simulink model "aerotest"  (R2021b)
settings: Solver=VariableStepAuto  StartTime=0.0  StopTime=10.0  RelTol=1e-3
undefined symbols (not defined in the file or in its folder): admireDB
libraries: simulink_extras x103, simulink x24, aerolibatmos2 x1
(part 2 of 13)

== system aerotest/YawMomentCoefficient/Subsystem ==
  mach_nd : Inport
  CymtotMR1 : Inport  Port=2
  CymtotMR2 : Inport  Port=3
  CymtotMR3 : Inport  Port=4
  CymtotMR4 : Inport  Port=5
  AND : Logic  IconShape=distinctive  AllPortsSameDT=off  OutDataTypeStr=boolean
  AND1 : Logic  IconShape=distinctive  AllPortsSameDT=off  OutDataTypeStr=boolean
  Compare To Constant1 : simulink/Logic and Bit Operations/Compare To Constant  relop=<=  const=0.4  OutDataTypeStr=boolean
  Compare To Constant2 : simulink/Logic and Bit Operations/Compare To Constant  relop=>  const=0.4  OutDataTypeStr=boolean
  Compare To Constant3 : simulink/Logic and Bit Operations/Compare To Constant  relop=<  const=0.5  OutDataTypeStr=boolean
  Compare To Constant4 : simulink/Logic and Bit Operations/Compare To Constant  relop=<=  const=1.4  OutDataTypeStr=boolean
  Compare To Constant5 : simulink/Logic and Bit Operations/Compare To Constant  relop=>=  const=0.5  OutDataTypeStr=boolean
  Switch : Switch  Criteria=u2 ~= 0
  Switch1 : Switch  Criteria=u2 ~= 0
  Switch2 : Switch  Criteria=u2 ~= 0
  Cymtot : Outport
  wires:
  Compare To Constant5/1 -> AND1/1
  Compare To Constant4/1 -> AND1/2
  AND1/1 -> Switch2/2
  CymtotMR4/1 -> Switch2/3
  CymtotMR3/1 -> Switch2/1
  Switch/1 -> Cymtot/1
  Switch2/1 -> Switch1/3
  CymtotMR2/1 -> Switch1/1
  Switch1/1 -> Switch/3
  CymtotMR1/1 -> Switch/1
  AND/1 -> Switch1/2
  Compare To Constant3/1 -> AND/2
  Compare To Constant2/1 -> AND/1
  Compare To Constant1/1 -> Switch/2
  mach_nd/1 -> Compare To Constant1/1, Compare To Constant3/1, Compare To Constant4/1, Compare To Constant5/1, Compare To Constant2/1

== system aerotest/CentripetalForceCoefficient/MachRegion1/Ccbcai ==
  in_bus : Inport
  Bus Selector : BusSelector  OutputSignals=AeroIn_Bus.cai,AeroIn_Bus.angleOfAttack_deg,AeroIn_Bus.angleOfSideslip_deg
  Ccbcai_ : Subsystem
  Ccbcai : Outport
  wires:
  Bus Selector/3 -> Ccbcai_/3(angleOfSideslip_deg)  "<angleOfSideslip_deg>"
  Bus Selector/2 -> Ccbcai_/2(angleOfAttack_deg)  "<angleOfAttack_deg>"
  in_bus/1 -> Bus Selector/1  "in_bus"
  Ccbcai_/1(Ccbcai) -> Ccbcai/1
  Bus Selector/1 -> Ccbcai_/1(CAI)  "<cai>"

== system aerotest/CentripetalForceCoefficient/MachRegion1/Ccbde ==
  in_bus : Inport
  Bus Selector : BusSelector  OutputSignals=AeroIn_Bus.angleOfSideslip_deg,AeroIn_Bus.dEI,AeroIn_Bus.angleOfAttack_deg,eieff,AeroIn_Bus.dEY,eoeff
  Ccbde_ : Subsystem
  Ccbde : Outport
  wires:
  Bus Selector/6 -> Ccbde_/6(eoeff)  "<eoeff>"
  Bus Selector/5 -> Ccbde_/5(dEY)  "<dEY>"
  Bus Selector/4 -> Ccbde_/4(eieff)  "<eieff>"
  Bus Selector/3 -> Ccbde_/3(angleOfAttack_deg)  "<angleOfAttack_deg>"
  Bus Selector/2 -> Ccbde_/2(dEI)  "<dEI>"
  Bus Selector/1 -> Ccbde_/1(angleOfSideslip_deg)  "<angleOfSideslip_deg>"
  Ccbde_/1(Ccbde) -> Ccbde/1
  in_bus/1 -> Bus Selector/1  "in_bus"

== system aerotest/CentripetalForceCoefficient/MachRegion1/Ccbdle ==
  in_bus : Inport
  Bus Selector : BusSelector  OutputSignals=AeroIn_Bus.lef_deg,AeroIn_Bus.angleOfSideslip_deg,AeroIn_Bus.angleOfAttack_deg
  Ccbdle_ : Subsystem
  Ccbdle : Outport
  wires:
  Bus Selector/3 -> Ccbdle_/3(angleOfAttack_deg)  "<angleOfAttack_deg>"
  Bus Selector/2 -> Ccbdle_/2(angleOfSideslip_deg)  "<angleOfSideslip_deg>"
  Bus Selector/1 -> Ccbdle_/1(dLE)  "<lef_deg>"
  Ccbdle_/1(Ccbdle) -> Ccbdle/1
  in_bus/1 -> Bus Selector/1  "in_bus"

== system aerotest/CentripetalForceCoefficient/MachRegion1/Ccbdn ==
  in_bus : Inport
  Bus Selector : BusSelector  OutputSignals=AeroIn_Bus.angleOfSideslip_deg,AeroIn_Bus.dN,AeroIn_Bus.angleOfAttack_deg
  Ccbdn_ : Subsystem
  Ccbdn : Outport
  wires:
  Bus Selector/2 -> Ccbdn_/2(dN)  "<dN>"
  Bus Selector/1 -> Ccbdn_/1(angleOfSideslip_deg)  "<angleOfSideslip_deg>"
  Bus Selector/3 -> Ccbdn_/3(angleOfAttack_deg)  "<angleOfAttack_deg>"
  in_bus/1 -> Bus Selector/1  "in_bus"
  Ccbdn_/1(Ccbdn) -> Ccbdn/1

== system aerotest/CentripetalForceCoefficient/MachRegion1/Ccbeta ==
  in_bus : Inport
  Bus Selector : BusSelector  OutputSignals=AeroIn_Bus.angleOfSideslip_deg,AeroIn_Bus.angleOfAttack_deg,AeroIn_Bus.qacorr,AeroIn_Bus.mach_nd
  Ccbeta_ : Subsystem
  Ccbeta : Outport
  wires:
  Ccbeta_/1(Ccbeta) -> Ccbeta/1
  Bus Selector/4 -> Ccbeta_/4(mach_nd)  "<mach_nd>"
  Bus Selector/3 -> Ccbeta_/3(qacorr)  "<qacorr>"
  Bus Selector/2 -> Ccbeta_/2(angleOfAttack_deg)  "<angleOfAttack_deg>"
  Bus Selector/1 -> Ccbeta_/1(angleOfSideslip_deg)  "<angleOfSideslip_deg>"
  in_bus/1 -> Bus Selector/1  "in_bus"

== system aerotest/CentripetalForceCoefficient/MachRegion1/Ccbetad ==
  in_bus : Inport
  Bus Selector : BusSelector  OutputSignals=AeroIn_Bus.angleOfAttack_deg,AeroIn_Bus.betad
  Ccbetad_ : Subsystem
  Ccbetad : Outport
  wires:
  Bus Selector/2 -> Ccbetad_/2(betad)  "<betad>"
  Bus Selector/1 -> Ccbetad_/1(angleOfAttack_deg)  "<angleOfAttack_deg>"
  in_bus/1 -> Bus Selector/1  "in_bus"
  Ccbetad_/1(Ccbetad) -> Ccbetad/1

== system aerotest/CentripetalForceCoefficient/MachRegion1/Ccblg ==
  in_bus : Inport
  Bus Selector : BusSelector  OutputSignals=AeroIn_Bus.lg_bool,AeroIn_Bus.angleOfAttack_deg,AeroIn_Bus.angleOfSideslip_deg
  Ccblg_ : Subsystem
  Ccblg : Outport
  wires:
  Bus Selector/1 -> Ccblg_/1(dLG)  "<lg_bool>"
  Bus Selector/3 -> Ccblg_/3(angleOfSideslip_deg)  "<angleOfSideslip_deg>"
  Bus Selector/2 -> Ccblg_/2(angleOfAttack_deg)  "<angleOfAttack_deg>"
  in_bus/1 -> Bus Selector/1  "in_bus"
  Ccblg_/1(Ccblg) -> Ccblg/1

== system aerotest/CentripetalForceCoefficient/MachRegion1/Ccdai ==
  in_bus : Inport
  Bus Selector : BusSelector  OutputSignals=AeroIn_Bus.dAI,AeroIn_Bus.angleOfAttack_deg,AeroIn_Bus.dEI,eieff,AeroIn_Bus.qacorr,AeroIn_Bus.mach_nd
  Ccdai_ : Subsystem
  Ccdai : Outport
  wires:
  Bus Selector/1 -> Ccdai_/1(dAI)  "<dAI>"
  Bus Selector/2 -> Ccdai_/2(angleOfAttack_deg)  "<angleOfAttack_deg>"
  Bus Selector/3 -> Ccdai_/3(dEI)  "<dEI>"
  Bus Selector/4 -> Ccdai_/4(eieff)  "<eieff>"
  Bus Selector/5 -> Ccdai_/5(qacorr)  "<qacorr>"
  Bus Selector/6 -> Ccdai_/6(mach_nd)  "<mach_nd>"
  in_bus/1 -> Bus Selector/1  "in_bus"
  Ccdai_/1(Ccdai) -> Ccdai/1

== system aerotest/CentripetalForceCoefficient/MachRegion1/Ccdaib ==
  in_bus : Inport
  Bus Selector : BusSelector  OutputSignals=AeroIn_Bus.angleOfAttack_deg,AeroIn_Bus.dAI,AeroIn_Bus.angleOfSideslip_deg,eieff
  Ccdaib_ : Subsystem
  Ccdaib : Outport
  wires:
  Bus Selector/4 -> Ccdaib_/4(eieff)  "<eieff>"
  Bus Selector/3 -> Ccdaib_/3(angleOfSideslip_deg)  "<angleOfSideslip_deg>"
  Bus Selector/1 -> Ccdaib_/1(angleOfAttack_deg)  "<angleOfAttack_deg>"
  Bus Selector/2 -> Ccdaib_/2(dAI)  "<dAI>"
  Ccdaib_/1(Ccdaib) -> Ccdaib/1
  in_bus/1 -> Bus Selector/1  "in_bus"

== system aerotest/CentripetalForceCoefficient/MachRegion1/Ccday ==
  in_bus : Inport
  Bus Selector : BusSelector  OutputSignals=AeroIn_Bus.dAY,AeroIn_Bus.angleOfAttack_deg,AeroIn_Bus.dEY,eoeff,AeroIn_Bus.qacorr,AeroIn_Bus.mach_nd
  Ccday_ : Subsystem
  Ccday : Outport
  wires:
  Ccday_/1(Ccday) -> Ccday/1
  in_bus/1 -> Bus Selector/1  "in_bus"
  Bus Selector/6 -> Ccday_/6(mach_nd)  "<mach_nd>"
  Bus Selector/5 -> Ccday_/5(qacorr)  "<qacorr>"
  Bus Selector/4 -> Ccday_/4(eoeff)  "<eoeff>"
  Bus Selector/3 -> Ccday_/3(dEY)  "<dEY>"
  Bus Selector/2 -> Ccday_/2(angleOfAttack_deg)  "<angleOfAttack_deg>"
  Bus Selector/1 -> Ccday_/1(dAY)  "<dAY>"

== system aerotest/CentripetalForceCoefficient/MachRegion1/Ccdayb ==
  in_bus : Inport
  Bus Selector : BusSelector  OutputSignals=AeroIn_Bus.angleOfAttack_deg,AeroIn_Bus.dAY,AeroIn_Bus.angleOfSideslip_deg,eoeff
  Ccdayb_ : Subsystem
  Ccdayb : Outport
  wires:
  in_bus/1 -> Bus Selector/1  "in_bus"
  Ccdayb_/1(Ccdayb) -> Ccdayb/1
  Bus Selector/2 -> Ccdayb_/2(dAY)  "<dAY>"
  Bus Selector/1 -> Ccdayb_/1(angleOfAttack_deg)  "<angleOfAttack_deg>"
  Bus Selector/3 -> Ccdayb_/3(angleOfSideslip_deg)  "<angleOfSideslip_deg>"
  Bus Selector/4 -> Ccdayb_/4(eoeff)  "<eoeff>"

== system aerotest/CentripetalForceCoefficient/MachRegion1/Ccdna ==
  in_bus : Inport
  Bus Selector : BusSelector  OutputSignals=AeroIn_Bus.dNE,AeroIn_Bus.angleOfAttack_deg,AeroIn_Bus.dNA
  Ccdna_ : Subsystem
  Ccdna : Outport
  wires:
  Bus Selector/3 -> Ccdna_/3(dNA)  "<dNA>"
  Bus Selector/1 -> Ccdna_/1(dNE)  "<dNE>"
  Bus Selector/2 -> Ccdna_/2(angleOfAttack_deg)  "<angleOfAttack_deg>"
  Ccdna_/1(Ccdna) -> Ccdna/1
  in_bus/1 -> Bus Selector/1  "in_bus"

== system aerotest/CentripetalForceCoefficient/MachRegion1/Ccdr ==
  in_bus : Inport
  Bus Selector : BusSelector  OutputSignals=AeroIn_Bus.angleOfAttack_deg,AeroIn_Bus.rud_deg,AeroIn_Bus.angleOfSideslip_deg,AeroIn_Bus.qacorr,AeroIn_Bus.mach_nd
  Ccdr_ : Subsystem
  Ccdr : Outport
  wires:
  Ccdr_/1(Ccdr) -> Ccdr/1
  Bus Selector/1 -> Ccdr_/1(angleOfAttack_deg)  "<angleOfAttack_deg>"
  Bus Selector/2 -> Ccdr_/2(dR)  "<rud_deg>"
  Bus Selector/3 -> Ccdr_/3(angleOfSideslip_deg)  "<angleOfSideslip_deg>"
  Bus Selector/4 -> Ccdr_/4(qacorr)  "<qacorr>"
  Bus Selector/5 -> Ccdr_/5(mach_nd)  "<mach_nd>"
  in_bus/1 -> Bus Selector/1  "in_bus"

== system aerotest/CentripetalForceCoefficient/MachRegion1/Ccp ==
  in_bus : Inport
  Bus Selector : BusSelector  OutputSignals=AeroIn_Bus.angleOfAttack_deg,AeroIn_Bus.pc
  Ccp_ : Subsystem
  Ccp : Outport
  wires:
  Ccp_/1(Ccp) -> Ccp/1
  in_bus/1 -> Bus Selector/1  "in_bus"
  Bus Selector/1 -> Ccp_/1(angleOfAttack_deg)  "<angleOfAttack_deg>"
  Bus Selector/2 -> Ccp_/2(pc)  "<pc>"

== system aerotest/CentripetalForceCoefficient/MachRegion1/Ccpbeta ==
  in_bus : Inport
  Bus Selector : BusSelector  OutputSignals=AeroIn_Bus.angleOfSideslip_deg,AeroIn_Bus.pc,AeroIn_Bus.angleOfAttack_deg
  Ccpbeta_ : Subsystem
  Ccpbeta : Outport
  wires:
  Bus Selector/3 -> Ccpbeta_/3(angleOfAttack_deg)  "<angleOfAttack_deg>"
  Bus Selector/1 -> Ccpbeta_/1(angleOfSideslip_deg)  "<angleOfSideslip_deg>"
  Bus Selector/2 -> Ccpbeta_/2(pc)  "<pc>"
  in_bus/1 -> Bus Selector/1  "in_bus"
  Ccpbeta_/1(Ccpbeta) -> Ccpbeta/1

== system aerotest/CentripetalForceCoefficient/MachRegion1/Ccr ==
  in_bus : Inport
  Bus Selector : BusSelector  OutputSignals=AeroIn_Bus.dN,AeroIn_Bus.angleOfAttack_deg,AeroIn_Bus.rc
  Ccr_ : Subsystem
  Ccr : Outport
  wires:
  Bus Selector/1 -> Ccr_/1(dN)  "<dN>"
  Bus Selector/3 -> Ccr_/3(rc)  "<rc>"
  Bus Selector/2 -> Ccr_/2(angleOfAttack_deg)  "<angleOfAttack_deg>"
  Ccr_/1(Ccr) -> Ccr/1
  in_bus/1 -> Bus Selector/1  "in_bus"

== system aerotest/CentripetalForceCoefficient/MachRegion1/Ccrbeta ==
  in_bus : Inport
  Bus Selector : BusSelector  OutputSignals=AeroIn_Bus.angleOfSideslip_deg,AeroIn_Bus.angleOfAttack_deg,AeroIn_Bus.rc
  Ccrbeta_ : Subsystem
  Ccrbeta : Outport
  wires:
  Bus Selector/3 -> Ccrbeta_/3(rc)  "<rc>"
  Bus Selector/1 -> Ccrbeta_/1(angleOfSideslip_deg)  "<angleOfSideslip_deg>"
  Bus Selector/2 -> Ccrbeta_/2(angleOfAttack_deg)  "<angleOfAttack_deg>"
  in_bus/1 -> Bus Selector/1  "in_bus"
  Ccrbeta_/1(Ccrbeta) -> Ccrbeta/1

== system aerotest/CentripetalForceCoefficient/MachRegion1/eoeff1 ==
  AeroIn_Bus : Inport
  Bus Selector : BusSelector  OutputSignals=mach_nd
  CCDAYOD_M : Lookup_n-D  NumberOfTableDimensions=1  BreakpointsForDimension1=admireDB.aerodata_asym_ext.CCDAYOD.breakpoints.M  BreakpointsForDimension3=[5, 7]  Table=admireDB.aerodata_asym_ext.CCDAYOD.newTable  ExtrapMethod=Clip  InternalRulePriority=Speed  RndMeth=Simplest  InputSameDT=on
  Constant : Constant
  Sum : Sum  Inputs=-+|
  eoeff : Outport
  eieff : Outport  Port=2
  wires:
  Sum/1 -> eieff/1
  CCDAYOD_M/1 -> eoeff/1, Sum/1
  Constant/1 -> Sum/2
  Bus Selector/1 -> CCDAYOD_M/1  "<mach_nd>"
  AeroIn_Bus/1 -> Bus Selector/1

== system aerotest/CentripetalForceCoefficient/MachRegion2/Ccbcai ==
  in_bus : Inport
  Bus Selector : BusSelector  OutputSignals=AeroIn_Bus.cai,AeroIn_Bus.angleOfAttack_deg,AeroIn_Bus.angleOfSideslip_deg
  Ccbcai_ : Subsystem
  Ccbcai : Outport
  wires:
  Bus Selector/1 -> Ccbcai_/1(cai)  "<cai>"
  Bus Selector/3 -> Ccbcai_/3(angleOfSideslip_deg)  "<angleOfSideslip_deg>"
  Bus Selector/2 -> Ccbcai_/2(angleOfAttack_deg)  "<angleOfAttack_deg>"
  in_bus/1 -> Bus Selector/1  "in_bus"
  Ccbcai_/1(Ccbcai) -> Ccbcai/1

== system aerotest/CentripetalForceCoefficient/MachRegion2/Ccbde ==
  in_bus : Inport
  Bus Selector : BusSelector  OutputSignals=AeroIn_Bus.angleOfAttack_deg,AeroIn_Bus.dEI,AeroIn_Bus.angleOfSideslip_deg,eieff,AeroIn_Bus.dEY,eoeff
  Ccbde_ : Subsystem
  Ccbde : Outport
  wires:
  Bus Selector/1 -> Ccbde_/1(angleOfAttack_deg)  "<angleOfAttack_deg>"
  Bus Selector/2 -> Ccbde_/2(dEI)  "<dEI>"
  Bus Selector/3 -> Ccbde_/3(angleOfSideslip_deg)  "<angleOfSideslip_deg>"
  Bus Selector/4 -> Ccbde_/4(eieff)  "<eieff>"
  Bus Selector/5 -> Ccbde_/5(dEY)  "<dEY>"
  Bus Selector/6 -> Ccbde_/6(eoeff)  "<eoeff>"
  Ccbde_/1(Ccbde) -> Ccbde/1
  in_bus/1 -> Bus Selector/1  "in_bus"

== system aerotest/CentripetalForceCoefficient/MachRegion2/Ccbdle ==
  in_bus : Inport
  Bus Selector : BusSelector  OutputSignals=AeroIn_Bus.angleOfAttack_deg,AeroIn_Bus.angleOfSideslip_deg,AeroIn_Bus.lef_deg,AeroIn_Bus.tflow,AeroIn_Bus.tfhigh
  Ccbdle_ : Subsystem
  Ccbdle : Outport
  wires:
  Bus Selector/5 -> Ccbdle_/5(tfhigh)  "<tfhigh>"
  Bus Selector/4 -> Ccbdle_/4(tflow)  "<tflow>"
  Bus Selector/3 -> Ccbdle_/3(dLE)  "<lef_deg>"
  Bus Selector/2 -> Ccbdle_/2(angleOfSideslip_deg)  "<angleOfSideslip_deg>"
  Bus Selector/1 -> Ccbdle_/1(angleOfAttack_deg)  "<angleOfAttack_deg>"
  Ccbdle_/1(Ccbdle) -> Ccbdle/1
  in_bus/1 -> Bus Selector/1  "in_bus"

== system aerotest/CentripetalForceCoefficient/MachRegion2/Ccbdn ==
  in_bus : Inport
  Bus Selector : BusSelector  OutputSignals=AeroIn_Bus.angleOfAttack_deg,AeroIn_Bus.dN,AeroIn_Bus.angleOfSideslip_deg
  Ccbdn_ : Subsystem
  Ccbdn : Outport
  wires:
  Bus Selector/1 -> Ccbdn_/1(angleOfAttack_deg)  "<angleOfAttack_deg>"
  Bus Selector/2 -> Ccbdn_/2(dN)  "<dN>"
  Bus Selector/3 -> Ccbdn_/3(angleOfSideslip_deg)  "<angleOfSideslip_deg>"
  in_bus/1 -> Bus Selector/1  "in_bus"
  Ccbdn_/1(Ccbdn) -> Ccbdn/1

== system aerotest/CentripetalForceCoefficient/MachRegion2/Ccbeta ==
  in_bus : Inport
  Bus Selector : BusSelector  OutputSignals=AeroIn_Bus.angleOfSideslip_deg,AeroIn_Bus.angleOfAttack_deg,AeroIn_Bus.tflow,AeroIn_Bus.tfhigh,AeroIn_Bus.qacorr,AeroIn_Bus.mach_nd
  Ccbeta_ : Subsystem
  Ccbeta : Outport
  wires:
  Bus Selector/6 -> Ccbeta_/6(mach_nd)  "<mach_nd>"
  Bus Selector/5 -> Ccbeta_/5(qacorr)  "<qacorr>"
  Bus Selector/4 -> Ccbeta_/4(tfhigh)  "<tfhigh>"
  Bus Selector/3 -> Ccbeta_/3(tflow)  "<tflow>"
  Bus Selector/2 -> Ccbeta_/2(angleOfAttack_deg)  "<angleOfAttack_deg>"
  Bus Selector/1 -> Ccbeta_/1(angleOfSideslip_deg)  "<angleOfSideslip_deg>"
  Ccbeta_/1(CCbeta) -> Ccbeta/1
  in_bus/1 -> Bus Selector/1  "in_bus"

== system aerotest/CentripetalForceCoefficient/MachRegion2/Ccbetad ==
  in_bus : Inport
  Bus Selector : BusSelector  OutputSignals=AeroIn_Bus.angleOfAttack_deg,AeroIn_Bus.tflow,AeroIn_Bus.betad,AeroIn_Bus.tfhigh
  CCbetad_ : Subsystem
  Ccbetad : Outport
  wires:
  Bus Selector/4 -> CCbetad_/4(tfhigh)  "<tfhigh>"
  Bus Selector/3 -> CCbetad_/3(betad)  "<betad>"
  Bus Selector/1 -> CCbetad_/1(angleOfAttack_deg)  "<angleOfAttack_deg>"
  Bus Selector/2 -> CCbetad_/2(tflow)  "<tflow>"
  CCbetad_/1(CCbetad) -> Ccbetad/1
  in_bus/1 -> Bus Selector/1  "in_bus"

== system aerotest/CentripetalForceCoefficient/MachRegion2/Ccblg ==
  in_bus : Inport
  Bus Selector : BusSelector  OutputSignals=AeroIn_Bus.lg_bool,AeroIn_Bus.angleOfAttack_deg,AeroIn_Bus.angleOfSideslip_deg
  Ccblg_ : Subsystem
  Ccblg : Outport
  wires:
  Bus Selector/1 -> Ccblg_/1(ldg)  "<lg_bool>"
  Bus Selector/3 -> Ccblg_/3(angleOfSideslip_deg)  "<angleOfSideslip_deg>"
  Bus Selector/2 -> Ccblg_/2(angleOfAttack_deg)  "<angleOfAttack_deg>"
  in_bus/1 -> Bus Selector/1  "in_bus"
  Ccblg_/1(Ccblg) -> Ccblg/1

== system aerotest/CentripetalForceCoefficient/MachRegion2/Ccdai ==
  in_bus : Inport
  Bus Selector : BusSelector  OutputSignals=AeroIn_Bus.dAI,AeroIn_Bus.angleOfAttack_deg,AeroIn_Bus.dEI,AeroIn_Bus.qacorr,AeroIn_Bus.mach_nd,AeroIn_Bus.tflow,AeroIn_Bus.tfhigh,eieff
  Ccdai_ : Subsystem
  Ccdai : Outport
  wires:
  Bus Selector/8 -> Ccdai_/8(eieff)  "<eieff>"
  Bus Selector/7 -> Ccdai_/7(tfhigh)  "<tfhigh>"
  Bus Selector/6 -> Ccdai_/6(tflow)  "<tflow>"
  Bus Selector/5 -> Ccdai_/5(mach_nd)  "<mach_nd>"
  Bus Selector/4 -> Ccdai_/4(qacorr)  "<qacorr>"
  Bus Selector/3 -> Ccdai_/3(dEI)  "<dEI>"
  Bus Selector/2 -> Ccdai_/2(angleOfAttack_deg)  "<angleOfAttack_deg>"
  Bus Selector/1 -> Ccdai_/1(dAI)  "<dAI>"
  in_bus/1 -> Bus Selector/1  "in_bus"
  Ccdai_/1(Ccdai) -> Ccdai/1

== system aerotest/CentripetalForceCoefficient/MachRegion2/Ccdaib ==
  in_bus : Inport
  Bus Selector : BusSelector  OutputSignals=AeroIn_Bus.angleOfAttack_deg,AeroIn_Bus.dAI,AeroIn_Bus.angleOfSideslip_deg,AeroIn_Bus.tflow,eieff
  Ccdaib_ : Subsystem
  Ccdaib : Outport
  wires:
  Bus Selector/5 -> Ccdaib_/5(eieff)  "<eieff>"
  Bus Selector/4 -> Ccdaib_/4(tflow)  "<tflow>"
  Bus Selector/3 -> Ccdaib_/3(angleOfSideslip_deg)  "<angleOfSideslip_deg>"
  Bus Selector/2 -> Ccdaib_/2(dAI)  "<dAI>"
  Bus Selector/1 -> Ccdaib_/1(angleOfAttack_deg)  "<angleOfAttack_deg>"
  Ccdaib_/1(Ccdaib) -> Ccdaib/1
  in_bus/1 -> Bus Selector/1  "in_bus"

== system aerotest/CentripetalForceCoefficient/MachRegion2/Ccday ==
  in_bus : Inport
  Bus Selector : BusSelector  OutputSignals=AeroIn_Bus.dAY,AeroIn_Bus.angleOfAttack_deg,AeroIn_Bus.dEY,AeroIn_Bus.qacorr,AeroIn_Bus.mach_nd,AeroIn_Bus.tflow,AeroIn_Bus.tfhigh,eoeff
  Ccday_ : Subsystem
  Ccday : Outport
  wires:
  Bus Selector/8 -> Ccday_/8(eoeff)  "<eoeff>"
  Bus Selector/7 -> Ccday_/7(tfhigh)  "<tfhigh>"
  Bus Selector/6 -> Ccday_/6(tflow)  "<tflow>"
  Bus Selector/5 -> Ccday_/5(mach_nd)  "<mach_nd>"
  Bus Selector/4 -> Ccday_/4(qacorr)  "<qacorr>"
  Bus Selector/3 -> Ccday_/3(dEY)  "<dEY>"
  Bus Selector/2 -> Ccday_/2(angleOfAttack_deg)  "<angleOfAttack_deg>"
  Bus Selector/1 -> Ccday_/1(dAY)  "<dAY>"
  in_bus/1 -> Bus Selector/1  "in_bus"
  Ccday_/1(Ccday) -> Ccday/1

== system aerotest/CentripetalForceCoefficient/MachRegion2/Ccdayb ==
  in_bus : Inport
  Bus Selector : BusSelector  OutputSignals=AeroIn_Bus.angleOfAttack_deg,AeroIn_Bus.dAY,AeroIn_Bus.angleOfSideslip_deg,AeroIn_Bus.tflow,eoeff
  Ccdayb_ : Subsystem
  Ccdayb : Outport
  wires:
  Bus Selector/1 -> Ccdayb_/1(angleOfAttack_deg)  "<angleOfAttack_deg>"
  Bus Selector/2 -> Ccdayb_/2(dAY)  "<dAY>"
  Bus Selector/3 -> Ccdayb_/3(angleOfSideslip_deg)  "<angleOfSideslip_deg>"
  Bus Selector/4 -> Ccdayb_/4(tflow)  "<tflow>"
  Bus Selector/5 -> Ccdayb_/5(eoeff)  "<eoeff>"
  Ccdayb_/1(Ccdaib) -> Ccdayb/1
  in_bus/1 -> Bus Selector/1  "in_bus"

== system aerotest/CentripetalForceCoefficient/MachRegion2/Ccdna ==
  in_bus : Inport
  Bus Selector : BusSelector  OutputSignals=AeroIn_Bus.dNE,AeroIn_Bus.angleOfAttack_deg,AeroIn_Bus.tflow,AeroIn_Bus.tfhigh,AeroIn_Bus.dNA
  Ccdna_ : Subsystem
  Ccdna : Outport
  wires:
  Bus Selector/5 -> Ccdna_/5(dNA)  "<dNA>"
  Bus Selector/4 -> Ccdna_/4(tfhigh)  "<tfhigh>"
  Bus Selector/3 -> Ccdna_/3(tflow)  "<tflow>"
  Bus Selector/2 -> Ccdna_/2(angleOfAttack_deg)  "<angleOfAttack_deg>"
  Bus Selector/1 -> Ccdna_/1(dNE)  "<dNE>"
  in_bus/1 -> Bus Selector/1  "in_bus"
  Ccdna_/1(Ccdna) -> Ccdna/1

== system aerotest/CentripetalForceCoefficient/MachRegion2/Ccdr ==
  in_bus : Inport
  Bus Selector : BusSelector  OutputSignals=AeroIn_Bus.angleOfAttack_deg,AeroIn_Bus.rud_deg,AeroIn_Bus.angleOfSideslip_deg,AeroIn_Bus.tflow,AeroIn_Bus.tfhigh,AeroIn_Bus.qacorr,AeroIn_Bus.mach_nd
  Ccdr_ : Subsystem
  Ccdr : Outport
  wires:
  Bus Selector/7 -> Ccdr_/7(mach_nd)  "<mach_nd>"
  Bus Selector/6 -> Ccdr_/6(qacorr)  "<qacorr>"
  Bus Selector/5 -> Ccdr_/5(tfhigh)  "<tfhigh>"
  Bus Selector/4 -> Ccdr_/4(tflow)  "<tflow>"
  Bus Selector/3 -> Ccdr_/3(angleOfSideslip_deg)  "<angleOfSideslip_deg>"
  Bus Selector/2 -> Ccdr_/2(dR)  "<rud_deg>"
  Bus Selector/1 -> Ccdr_/1(angleOfAttack_deg)  "<angleOfAttack_deg>"
  Ccdr_/1(Ccdr) -> Ccdr/1
  in_bus/1 -> Bus Selector/1  "in_bus"

== system aerotest/CentripetalForceCoefficient/MachRegion2/Ccp ==
  in_bus : Inport
  Bus Selector : BusSelector  OutputSignals=AeroIn_Bus.angleOfAttack_deg,AeroIn_Bus.tflow,AeroIn_Bus.pc,AeroIn_Bus.tfhigh
  Ccp_ : Subsystem
  Ccp : Outport
  wires:
  Bus Selector/4 -> Ccp_/4(tfhigh)  "<tfhigh>"
  Bus Selector/3 -> Ccp_/3(pc)  "<pc>"
  Bus Selector/1 -> Ccp_/1(angleOfAttack_deg)  "<angleOfAttack_deg>"
  Bus Selector/2 -> Ccp_/2(tflow)  "<tflow>"
  in_bus/1 -> Bus Selector/1  "in_bus"
  Ccp_/1(Ccp) -> Ccp/1

== system aerotest/CentripetalForceCoefficient/MachRegion2/Ccpbeta ==
  in_bus : Inport
  Bus Selector : BusSelector  OutputSignals=AeroIn_Bus.angleOfSideslip_deg,AeroIn_Bus.angleOfAttack_deg,AeroIn_Bus.tflow,AeroIn_Bus.pc
  Ccpbeta_ : Subsystem
  Ccpbeta : Outport
  wires:
  Bus Selector/4 -> Ccpbeta_/4(pc)  "<pc>"
  Bus Selector/3 -> Ccpbeta_/3(tflow)  "<tflow>"
  Bus Selector/2 -> Ccpbeta_/2(angleOfAttack_deg)  "<angleOfAttack_deg>"
  Bus Selector/1 -> Ccpbeta_/1(angleOfSideslip_deg)  "<angleOfSideslip_deg>"
  Ccpbeta_/1(Ccpbeta) -> Ccpbeta/1
  in_bus/1 -> Bus Selector/1  "in_bus"

== system aerotest/CentripetalForceCoefficient/MachRegion2/Ccr ==
  in_bus : Inport
  Bus Selector : BusSelector  OutputSignals=AeroIn_Bus.dN,AeroIn_Bus.angleOfAttack_deg,AeroIn_Bus.tflow,AeroIn_Bus.tfhigh,AeroIn_Bus.rc,AeroIn_Bus.mach_nd,AeroIn_Bus.qacorr
  Ccr_ : Subsystem
  Ccr : Outport
  wires:
  Bus Selector/7 -> Ccr_/7(qacorr)  "<qacorr>"
  Bus Selector/6 -> Ccr_/6(mach_nd)  "<mach_nd>"
  Bus Selector/5 -> Ccr_/5(rc)  "<rc>"
  Bus Selector/4 -> Ccr_/4(tfhigh)  "<tfhigh>"
  Bus Selector/3 -> Ccr_/3(tflow)  "<tflow>"
  Bus Selector/2 -> Ccr_/2(angleOfAttack_deg)  "<angleOfAttack_deg>"
  Bus Selector/1 -> Ccr_/1(dN)  "<dN>"
  in_bus/1 -> Bus Selector/1  "in_bus"
  Ccr_/1(Ccr) -> Ccr/1

== system aerotest/CentripetalForceCoefficient/MachRegion2/Ccrbeta ==
  in_bus : Inport
  Bus Selector : BusSelector  OutputSignals=AeroIn_Bus.angleOfSideslip_deg,AeroIn_Bus.angleOfAttack_deg,AeroIn_Bus.tflow,AeroIn_Bus.rc
  Ccrbeta_ : Subsystem
  Ccrbeta : Outport
  wires:
  Bus Selector/1 -> Ccrbeta_/1(angleOfSideslip_deg)  "<angleOfSideslip_deg>"
  Bus Selector/2 -> Ccrbeta_/2(angleOfAttack_deg)  "<angleOfAttack_deg>"
  Bus Selector/4 -> Ccrbeta_/4(rc)  "<rc>"
  Bus Selector/3 -> Ccrbeta_/3(tflow)  "<tflow>"
  Ccrbeta_/1(Ccrbeta) -> Ccrbeta/1
  in_bus/1 -> Bus Selector/1  "in_bus"

== system aerotest/CentripetalForceCoefficient/MachRegion2/eoeff1 ==
  AeroIn_Bus : Inport
  Bus Selector : BusSelector  OutputSignals=mach_nd
  CCDAYOD_M : Lookup_n-D  NumberOfTableDimensions=1  BreakpointsForDimension1=admireDB.aerodata_asym_ext.CCDAYOD.breakpoints.M  BreakpointsForDimension3=[5, 7]  Table=admireDB.aerodata_asym_ext.CCDAYOD.newTable  ExtrapMethod=Clip  InternalRulePriority=Speed  RndMeth=Simplest  InputSameDT=on
  Constant : Constant
  Sum : Sum  Inputs=-+|
  eoeff : Outport
  eieff : Outport  Port=2
  wires:
  Sum/1 -> eieff/1
  CCDAYOD_M/1 -> eoeff/1, Sum/1
  Constant/1 -> Sum/2
  Bus Selector/1 -> CCDAYOD_M/1  "<mach_nd>"
  AeroIn_Bus/1 -> Bus Selector/1

== system aerotest/CentripetalForceCoefficient/MachRegion3/Ccbcai ==
  in_bus : Inport
  Bus Selector : BusSelector  OutputSignals=AeroIn_Bus.cai,AeroIn_Bus.angleOfAttack_deg,AeroIn_Bus.angleOfSideslip_deg
  Ccbcai_ : Subsystem
  Ccbcai : Outport
  wires:
  Bus Selector/1 -> Ccbcai_/1(cai)  "<cai>"
  Bus Selector/3 -> Ccbcai_/3(angleOfSideslip_deg)  "<angleOfSideslip_deg>"
  Bus Selector/2 -> Ccbcai_/2(angleOfAttack_deg)  "<angleOfAttack_deg>"
  in_bus/1 -> Bus Selector/1  "in_bus"
  Ccbcai_/1(Ccbcai) -> Ccbcai/1

== system aerotest/CentripetalForceCoefficient/MachRegion3/Ccbde ==
  in_bus : Inport
  Bus Selector : BusSelector  OutputSignals=AeroIn_Bus.angleOfAttack_deg,AeroIn_Bus.dEI,AeroIn_Bus.angleOfSideslip_deg,AeroIn_Bus.dEY,eieff,eoeff,AeroIn_Bus.mach_nd
  Ccbde_ : Subsystem
  Ccbde : Outport
  wires:
  Bus Selector/7 -> Ccbde_/7(mach_nd)  "<mach_nd>"
  Bus Selector/6 -> Ccbde_/6(eoeff)  "<eoeff>"
  Bus Selector/5 -> Ccbde_/5(eieff)  "<eieff>"
  Bus Selector/4 -> Ccbde_/4(dEY)  "<dEY>"
  Bus Selector/3 -> Ccbde_/3(angleOfSideslip_deg)  "<angleOfSideslip_deg>"
  Bus Selector/2 -> Ccbde_/2(dEI)  "<dEI>"
  Bus Selector/1 -> Ccbde_/1(angleOfAttack_deg)  "<angleOfAttack_deg>"
  Ccbde_/1(Ccbde) -> Ccbde/1
  in_bus/1 -> Bus Selector/1  "in_bus"

== system aerotest/CentripetalForceCoefficient/MachRegion3/Ccbdle ==
  in_bus : Inport
  Bus Selector : BusSelector  OutputSignals=AeroIn_Bus.mach_nd,AeroIn_Bus.angleOfAttack_deg,AeroIn_Bus.angleOfSideslip_deg,AeroIn_Bus.lef_deg
  Ccbdle_ : Subsystem
  Ccbdle : Outport
  wires:
  Bus Selector/4 -> Ccbdle_/4(dLE)  "<lef_deg>"
  Bus Selector/3 -> Ccbdle_/3(angleOfSideslip_deg)  "<angleOfSideslip_deg>"
  Bus Selector/1 -> Ccbdle_/1(mach_nd)  "<mach_nd>"
  Bus Selector/2 -> Ccbdle_/2(angleOfAttack_deg)  "<angleOfAttack_deg>"
  Ccbdle_/1(Ccbdle) -> Ccbdle/1
  in_bus/1 -> Bus Selector/1  "in_bus"

== system aerotest/CentripetalForceCoefficient/MachRegion3/Ccbdn ==
  in_bus : Inport
  Bus Selector : BusSelector  OutputSignals=AeroIn_Bus.angleOfAttack_deg,AeroIn_Bus.dN,AeroIn_Bus.angleOfSideslip_deg
  Ccbdn_ : Subsystem
  Ccbdn : Outport
  wires:
  Bus Selector/3 -> Ccbdn_/3(angleOfSideslip_deg)  "<angleOfSideslip_deg>"
  Bus Selector/2 -> Ccbdn_/2(dN)  "<dN>"
  Bus Selector/1 -> Ccbdn_/1(angleOfAttack_deg)  "<angleOfAttack_deg>"
  in_bus/1 -> Bus Selector/1  "in_bus"
  Ccbdn_/1(Ccbdn) -> Ccbdn/1

== system aerotest/CentripetalForceCoefficient/MachRegion3/Ccbeta ==
  in_bus : Inport
  Bus Selector : BusSelector  OutputSignals=AeroIn_Bus.mach_nd,AeroIn_Bus.angleOfAttack_deg,AeroIn_Bus.angleOfSideslip_deg,AeroIn_Bus.qacorr
  Ccbeta_ : Subsystem
  Ccbeta : Outport
  wires:
  Bus Selector/1 -> Ccbeta_/1(mach_nd)  "<mach_nd>"
  Bus Selector/2 -> Ccbeta_/2(angleOfAttack_deg)  "<angleOfAttack_deg>"
  Bus Selector/3 -> Ccbeta_/3(angleOfSideslip_deg)  "<angleOfSideslip_deg>"
  Bus Selector/4 -> Ccbeta_/4(qacorr)  "<qacorr>"
  Ccbeta_/1(CCbeta) -> Ccbeta/1
  in_bus/1 -> Bus Selector/1  "in_bus"

== system aerotest/CentripetalForceCoefficient/MachRegion3/Ccbetad ==
  in_bus : Inport
  Bus Selector : BusSelector  OutputSignals=AeroIn_Bus.angleOfAttack_deg,AeroIn_Bus.mach_nd,AeroIn_Bus.betad
  Ccbetad_ : Subsystem
  Ccbetad : Outport
  wires:
  Bus Selector/1 -> Ccbetad_/1(angleOfAttack_deg)  "<angleOfAttack_deg>"
  Bus Selector/2 -> Ccbetad_/2(mach_nd)  "<mach_nd>"
  Bus Selector/3 -> Ccbetad_/3(betad)  "<betad>"
  Ccbetad_/1(CCbetad) -> Ccbetad/1
  in_bus/1 -> Bus Selector/1  "in_bus"

== system aerotest/CentripetalForceCoefficient/MachRegion3/Ccblg ==
  in_bus : Inport
  Bus Selector : BusSelector  OutputSignals=AeroIn_Bus.lg_bool,AeroIn_Bus.angleOfAttack_deg,AeroIn_Bus.angleOfSideslip_deg
  Ccblg_ : Subsystem
  Ccblg : Outport
  wires:
  Bus Selector/1 -> Ccblg_/1(ldg)  "<lg_bool>"
  Bus Selector/3 -> Ccblg_/3(angleOfSideslip_deg)  "<angleOfSideslip_deg>"
  Bus Selector/2 -> Ccblg_/2(angleOfAttack_deg)  "<angleOfAttack_deg>"
  in_bus/1 -> Bus Selector/1  "in_bus"
  Ccblg_/1(Ccblg) -> Ccblg/1

== system aerotest/CentripetalForceCoefficient/MachRegion3/Ccdai ==
  in_bus : Inport
  Bus Selector : BusSelector  OutputSignals=AeroIn_Bus.angleOfAttack_deg,AeroIn_Bus.dAI,AeroIn_Bus.mach_nd,AeroIn_Bus.dEI,eieff,AeroIn_Bus.qacorr
  Ccdai_ : Subsystem
  Ccdai : Outport
  wires:
  Bus Selector/6 -> Ccdai_/6(qacorr)  "<qacorr>"
  Bus Selector/5 -> Ccdai_/5(eieff)  "<eieff>"
  Bus Selector/4 -> Ccdai_/4(dEI)  "<dEI>"
  Bus Selector/3 -> Ccdai_/3(mach_nd)  "<mach_nd>"
  Bus Selector/1 -> Ccdai_/1(angleOfAttack_deg)  "<angleOfAttack_deg>"
  Bus Selector/2 -> Ccdai_/2(dAI)  "<dAI>"
  in_bus/1 -> Bus Selector/1  "in_bus"
  Ccdai_/1(Ccdai) -> Ccdai/1

== system aerotest/CentripetalForceCoefficient/MachRegion3/Ccdaib ==
  Constant : Constant  Value=0
  Ccdaib : Outport
  wires:
  Constant/1 -> Ccdaib/1

== system aerotest/CentripetalForceCoefficient/MachRegion3/Ccday ==
  in_bus : Inport
  Bus Selector : BusSelector  OutputSignals=AeroIn_Bus.angleOfAttack_deg,AeroIn_Bus.dAY,AeroIn_Bus.mach_nd,AeroIn_Bus.dEY,eoeff,AeroIn_Bus.qacorr
  Ccday_ : Subsystem
  Ccday : Outport
  wires:
  Ccday_/1(Ccday) -> Ccday/1
  in_bus/1 -> Bus Selector/1  "in_bus"
  Bus Selector/2 -> Ccday_/2(dAY)  "<dAY>"
  Bus Selector/1 -> Ccday_/1(angleOfAttack_deg)  "<angleOfAttack_deg>"
  Bus Selector/3 -> Ccday_/3(mach_nd)  "<mach_nd>"
  Bus Selector/4 -> Ccday_/4(dEY)  "<dEY>"
  Bus Selector/5 -> Ccday_/5(eoeff)  "<eoeff>"
  Bus Selector/6 -> Ccday_/6(qacorr)  "<qacorr>"

== system aerotest/CentripetalForceCoefficient/MachRegion3/Ccdayb ==
  Constant : Constant  Value=0
  Ccdayb : Outport
  wires:
  Constant/1 -> Ccdayb/1

== system aerotest/CentripetalForceCoefficient/MachRegion3/Ccdna ==
  in_bus : Inport
  Bus Selector : BusSelector  OutputSignals=AeroIn_Bus.angleOfAttack_deg,AeroIn_Bus.mach_nd,AeroIn_Bus.dNA
  Ccdna_ : Subsystem
  Ccdna : Outport
  wires:
  Bus Selector/1 -> Ccdna_/1(angleOfAttack_deg)  "<angleOfAttack_deg>"
  Bus Selector/3 -> Ccdna_/3(dNA)  "<dNA>"
  Bus Selector/2 -> Ccdna_/2(mach_nd)  "<mach_nd>"
  in_bus/1 -> Bus Selector/1  "in_bus"
  Ccdna_/1(Ccdna) -> Ccdna/1

== system aerotest/CentripetalForceCoefficient/MachRegion3/Ccdr ==
  in_bus : Inport
  Bus Selector : BusSelector  OutputSignals=AeroIn_Bus.angleOfAttack_deg,AeroIn_Bus.mach_nd,AeroIn_Bus.rud_deg,AeroIn_Bus.qacorr
  Ccdr_ : Subsystem
  Ccdr : Outport
  wires:
  Bus Selector/1 -> Ccdr_/1(angleOfAttack_deg)  "<angleOfAttack_deg>"
  Bus Selector/2 -> Ccdr_/2(mach_nd)  "<mach_nd>"
  Bus Selector/3 -> Ccdr_/3(dR)  "<rud_deg>"
  Bus Selector/4 -> Ccdr_/4(qacorr)  "<qacorr>"
  Ccdr_/1(Ccdr) -> Ccdr/1
  in_bus/1 -> Bus Selector/1  "in_bus"

== system aerotest/CentripetalForceCoefficient/MachRegion3/Ccp1 ==
  in_bus : Inport
  Bus Selector : BusSelector  OutputSignals=AeroIn_Bus.angleOfAttack_deg,AeroIn_Bus.mach_nd,AeroIn_Bus.pc
  Ccp_ : Subsystem
  Ccp : Outport
  wires:
  Bus Selector/1 -> Ccp_/1(angleOfAttack_deg)  "<angleOfAttack_deg>"
  Bus Selector/2 -> Ccp_/2(mach_nd)  "<mach_nd>"
  Bus Selector/3 -> Ccp_/3(pc)  "<pc>"
  in_bus/1 -> Bus Selector/1  "in_bus"
  Ccp_/1(Ccp) -> Ccp/1

== system aerotest/CentripetalForceCoefficient/MachRegion3/Ccpbeta ==
  Constant : Constant  Value=0
  Ccpbeta : Outport
  wires:
  Constant/1 -> Ccpbeta/1

== system aerotest/CentripetalForceCoefficient/MachRegion3/Ccr1 ==
  in_bus : Inport
  Bus Selector : BusSelector  OutputSignals=AeroIn_Bus.mach_nd,AeroIn_Bus.rc
  Ccr_ : Subsystem
  Ccr : Outport
  wires:
  Bus Selector/2 -> Ccr_/2(rc)  "<rc>"
  Bus Selector/1 -> Ccr_/1(mach_nd)  "<mach_nd>"
  in_bus/1 -> Bus Selector/1  "in_bus"
  Ccr_/1(Ccr) -> Ccr/1

== system aerotest/CentripetalForceCoefficient/MachRegion3/Ccrbeta ==
  Constant : Constant  Value=0
  Ccrbeta : Outport
  wires:
  Constant/1 -> Ccrbeta/1

== system aerotest/CentripetalForceCoefficient/MachRegion3/eoeff1 ==
  AeroIn_Bus : Inport
  Bus Selector : BusSelector  OutputSignals=mach_nd
  CCDAYOD_M : Lookup_n-D  NumberOfTableDimensions=1  BreakpointsForDimension1=admireDB.aerodata_asym_ext.CCDAYOD.breakpoints.M  BreakpointsForDimension3=[5, 7]  Table=admireDB.aerodata_asym_ext.CCDAYOD.newTable  ExtrapMethod=Clip  InternalRulePriority=Speed  RndMeth=Simplest  InputSameDT=on
  Constant : Constant
  Sum : Sum  Inputs=-+|
  eoeff : Outport
  eieff : Outport  Port=2
  wires:
  Sum/1 -> eieff/1
  CCDAYOD_M/1 -> eoeff/1, Sum/1
  Constant/1 -> Sum/2
  Bus Selector/1 -> CCDAYOD_M/1  "<mach_nd>"
  AeroIn_Bus/1 -> Bus Selector/1

== system aerotest/CentripetalForceCoefficient/MachRegion4/Ccbcai ==
  in_bus : Inport
  Bus Selector : BusSelector  OutputSignals=AeroIn_Bus.cai,AeroIn_Bus.angleOfAttack_deg,AeroIn_Bus.angleOfSideslip_deg
  Ccbcai_ : Subsystem
  Ccbcai : Outport
  wires:
  Bus Selector/1 -> Ccbcai_/1(cai)  "<cai>"
  Bus Selector/3 -> Ccbcai_/3(angleOfSideslip_deg)  "<angleOfSideslip_deg>"
  Bus Selector/2 -> Ccbcai_/2(angleOfAttack_deg)  "<angleOfAttack_deg>"
  in_bus/1 -> Bus Selector/1  "in_bus"
  Ccbcai_/1(Ccbcai) -> Ccbcai/1

== system aerotest/CentripetalForceCoefficient/MachRegion4/Ccbde ==
  in_bus : Inport
  Bus Selector : BusSelector  OutputSignals=AeroIn_Bus.angleOfAttack_deg,AeroIn_Bus.dEI,AeroIn_Bus.angleOfSideslip_deg,AeroIn_Bus.dEY,eieff,eoeff,AeroIn_Bus.mach_nd
  Ccbde_ : Subsystem
  Ccbde : Outport
  wires:
  Bus Selector/7 -> Ccbde_/7(mach_nd)  "<mach_nd>"
  Bus Selector/6 -> Ccbde_/6(eoeff)  "<eoeff>"
  Bus Selector/5 -> Ccbde_/5(eieff)  "<eieff>"
  Bus Selector/4 -> Ccbde_/4(dEY)  "<dEY>"
  Bus Selector/3 -> Ccbde_/3(angleOfSideslip_deg)  "<angleOfSideslip_deg>"
  Bus Selector/2 -> Ccbde_/2(dEI)  "<dEI>"
  Bus Selector/1 -> Ccbde_/1(angleOfAttack_deg)  "<angleOfAttack_deg>"
  Ccbde_/1(Ccbde) -> Ccbde/1
  in_bus/1 -> Bus Selector/1  "in_bus"

== system aerotest/CentripetalForceCoefficient/MachRegion4/Ccbdle ==
  in_bus : Inport
  Bus Selector : BusSelector  OutputSignals=AeroIn_Bus.mach_nd,AeroIn_Bus.angleOfAttack_deg,AeroIn_Bus.angleOfSideslip_deg,AeroIn_Bus.lef_deg
  Ccbdle_ : Subsystem
  Ccbdle : Outport
  wires:
  Bus Selector/4 -> Ccbdle_/4(dLE)  "<lef_deg>"
  Bus Selector/3 -> Ccbdle_/3(angleOfSideslip_deg)  "<angleOfSideslip_deg>"
  Bus Selector/1 -> Ccbdle_/1(mach_nd)  "<mach_nd>"
  Bus Selector/2 -> Ccbdle_/2(angleOfAttack_deg)  "<angleOfAttack_deg>"
  Ccbdle_/1(Ccbdle) -> Ccbdle/1
  in_bus/1 -> Bus Selector/1  "in_bus"

== system aerotest/CentripetalForceCoefficient/MachRegion4/Ccbdn ==
  in_bus : Inport
  Bus Selector : BusSelector  OutputSignals=AeroIn_Bus.angleOfAttack_deg,AeroIn_Bus.dN,AeroIn_Bus.angleOfSideslip_deg
  Ccbdn_ : Subsystem
  Ccbdn : Outport
  wires:
  Bus Selector/3 -> Ccbdn_/3(angleOfSideslip_deg)  "<angleOfSideslip_deg>"
  Bus Selector/2 -> Ccbdn_/2(dN)  "<dN>"
  Bus Selector/1 -> Ccbdn_/1(angleOfAttack_deg)  "<angleOfAttack_deg>"
  in_bus/1 -> Bus Selector/1  "in_bus"
  Ccbdn_/1(Ccbdn) -> Ccbdn/1

== system aerotest/CentripetalForceCoefficient/MachRegion4/Ccbeta ==
  in_bus : Inport
  Bus Selector : BusSelector  OutputSignals=AeroIn_Bus.mach_nd,AeroIn_Bus.angleOfAttack_deg,AeroIn_Bus.angleOfSideslip_deg,AeroIn_Bus.qacorr
  Ccbeta_ : Subsystem
  Ccbeta : Outport
  wires:
  Bus Selector/1 -> Ccbeta_/1(mach_nd)  "<mach_nd>"
  Bus Selector/2 -> Ccbeta_/2(angleOfAttack_deg)  "<angleOfAttack_deg>"
  Bus Selector/3 -> Ccbeta_/3(angleOfSideslip_deg)  "<angleOfSideslip_deg>"
  Bus Selector/4 -> Ccbeta_/4(qacorr)  "<qacorr>"
  Ccbeta_/1(CCbeta) -> Ccbeta/1
  in_bus/1 -> Bus Selector/1  "in_bus"

== system aerotest/CentripetalForceCoefficient/MachRegion4/Ccbetad ==
  in_bus : Inport
  Bus Selector : BusSelector  OutputSignals=AeroIn_Bus.angleOfAttack_deg,AeroIn_Bus.mach_nd,AeroIn_Bus.betad
  Ccbetad_ : Subsystem
  Ccbetad : Outport
  wires:
  Bus Selector/1 -> Ccbetad_/1(angleOfAttack_deg)  "<angleOfAttack_deg>"
  Bus Selector/2 -> Ccbetad_/2(mach_nd)  "<mach_nd>"
  Bus Selector/3 -> Ccbetad_/3(betad)  "<betad>"
  Ccbetad_/1(CCbetad) -> Ccbetad/1
  in_bus/1 -> Bus Selector/1  "in_bus"

== system aerotest/CentripetalForceCoefficient/MachRegion4/Ccblg ==
  in_bus : Inport
  Bus Selector : BusSelector  OutputSignals=AeroIn_Bus.lg_bool,AeroIn_Bus.angleOfAttack_deg,AeroIn_Bus.angleOfSideslip_deg
  Ccblg_ : Subsystem
  Ccblg : Outport
  wires:
  Bus Selector/1 -> Ccblg_/1(ldg)  "<lg_bool>"
  Bus Selector/3 -> Ccblg_/3(angleOfSideslip_deg)  "<angleOfSideslip_deg>"
  Bus Selector/2 -> Ccblg_/2(angleOfAttack_deg)  "<angleOfAttack_deg>"
  in_bus/1 -> Bus Selector/1  "in_bus"
  Ccblg_/1(Ccblg) -> Ccblg/1

== system aerotest/CentripetalForceCoefficient/MachRegion4/Ccdai ==
  in_bus : Inport
  Bus Selector : BusSelector  OutputSignals=AeroIn_Bus.dAI,AeroIn_Bus.angleOfAttack_deg,AeroIn_Bus.dEI,AeroIn_Bus.qacorr,eieff,AeroIn_Bus.mach_nd
  Ccdai_ : Subsystem
  Ccdai : Outport
  wires:
  Bus Selector/1 -> Ccdai_/1(dAI)  "<dAI>"
  Bus Selector/2 -> Ccdai_/2(angleOfAttack_deg)  "<angleOfAttack_deg>"
  Bus Selector/3 -> Ccdai_/3(dEI)  "<dEI>"
  Bus Selector/4 -> Ccdai_/4(qacorr)  "<qacorr>"
  Bus Selector/5 -> Ccdai_/5(eieff)  "<eieff>"
  Bus Selector/6 -> Ccdai_/6(mach_nd)  "<mach_nd>"
  in_bus/1 -> Bus Selector/1  "in_bus"
  Ccdai_/1(Ccdai) -> Ccdai/1

== system aerotest/CentripetalForceCoefficient/MachRegion4/Ccdaib ==
  Constant : Constant  Value=0
  Ccdaib : Outport
  wires:
  Constant/1 -> Ccdaib/1

== system aerotest/CentripetalForceCoefficient/MachRegion4/Ccday ==
  in_bus : Inport
  Bus Selector : BusSelector  OutputSignals=AeroIn_Bus.angleOfAttack_deg,AeroIn_Bus.dEY,AeroIn_Bus.mach_nd,AeroIn_Bus.qacorr,eoeff,AeroIn_Bus.dAY
  Ccday_ : Subsystem
  Ccday : Outport
  wires:
  Bus Selector/6 -> Ccday_/6(dAY)  "<dAY>"
  Bus Selector/5 -> Ccday_/5(eoeff)  "<eoeff>"
  Bus Selector/4 -> Ccday_/4(qacorr)  "<qacorr>"
  Bus Selector/3 -> Ccday_/3(mach_nd)  "<mach_nd>"
  Bus Selector/2 -> Ccday_/2(dEY)  "<dEY>"
  Bus Selector/1 -> Ccday_/1(angleOfAttack_deg)  "<angleOfAttack_deg>"
  Ccday_/1(Ccday) -> Ccday/1
  in_bus/1 -> Bus Selector/1  "in_bus"

== system aerotest/CentripetalForceCoefficient/MachRegion4/Ccdayb ==
  Constant : Constant  Value=0
  Ccdayb : Outport
  wires:
  Constant/1 -> Ccdayb/1

== system aerotest/CentripetalForceCoefficient/MachRegion4/Ccdna ==
  in_bus : Inport
  Bus Selector : BusSelector  OutputSignals=AeroIn_Bus.angleOfAttack_deg,AeroIn_Bus.mach_nd,AeroIn_Bus.dNA
  Ccdna_ : Subsystem
  Ccdna : Outport
  wires:
  Bus Selector/1 -> Ccdna_/1(angleOfAttack_deg)  "<angleOfAttack_deg>"
  Bus Selector/3 -> Ccdna_/3(dNA)  "<dNA>"
  Bus Selector/2 -> Ccdna_/2(mach_nd)  "<mach_nd>"
  in_bus/1 -> Bus Selector/1  "in_bus"
  Ccdna_/1(Ccdna) -> Ccdna/1

== system aerotest/CentripetalForceCoefficient/MachRegion4/Ccdr ==
  in_bus : Inport
  Bus Selector : BusSelector  OutputSignals=AeroIn_Bus.angleOfAttack_deg,AeroIn_Bus.mach_nd,AeroIn_Bus.rud_deg,AeroIn_Bus.qacorr
  Ccdr_ : Subsystem
  Ccdr : Outport
  wires:
  Bus Selector/1 -> Ccdr_/1(angleOfAttack_deg)  "<angleOfAttack_deg>"
  Bus Selector/2 -> Ccdr_/2(mach_nd)  "<mach_nd>"
  Bus Selector/3 -> Ccdr_/3(dR)  "<rud_deg>"
  Bus Selector/4 -> Ccdr_/4(qacorr)  "<qacorr>"
  Ccdr_/1(Ccdr) -> Ccdr/1
  in_bus/1 -> Bus Selector/1  "in_bus"

== system aerotest/CentripetalForceCoefficient/MachRegion4/Ccp ==
  in_bus : Inport
  Bus Selector : BusSelector  OutputSignals=AeroIn_Bus.angleOfAttack_deg,AeroIn_Bus.mach_nd,AeroIn_Bus.pc
  Ccp_ : Subsystem
  Ccp : Outport
  wires:
  Bus Selector/1 -> Ccp_/1(angleOfAttack_deg)  "<angleOfAttack_deg>"
  Bus Selector/2 -> Ccp_/2(mach_nd)  "<mach_nd>"
  Bus Selector/3 -> Ccp_/3(pc)  "<pc>"
  in_bus/1 -> Bus Selector/1  "in_bus"
  Ccp_/1(Ccp) -> Ccp/1

== system aerotest/CentripetalForceCoefficient/MachRegion4/Ccpbeta ==
  Constant : Constant  Value=0
  Ccpbeta : Outport
  wires:
  Constant/1 -> Ccpbeta/1

== system aerotest/CentripetalForceCoefficient/MachRegion4/Ccr ==
  in_bus : Inport
  Bus Selector : BusSelector  OutputSignals=AeroIn_Bus.mach_nd,AeroIn_Bus.qacorr,AeroIn_Bus.rc
  Ccr_ : Subsystem
  Ccr : Outport
  wires:
  Bus Selector/3 -> Ccr_/3(rc)  "<rc>"
  Bus Selector/2 -> Ccr_/2(qacorr)  "<qacorr>"
  Bus Selector/1 -> Ccr_/1(mach_nd)  "<mach_nd>"
  in_bus/1 -> Bus Selector/1  "in_bus"
  Ccr_/1(Ccr) -> Ccr/1

== system aerotest/CentripetalForceCoefficient/MachRegion4/Ccrbeta ==
  Constant : Constant  Value=0
  Ccrbeta : Outport
  wires:
  Constant/1 -> Ccrbeta/1

== system aerotest/CentripetalForceCoefficient/MachRegion4/eoeff ==
  AeroIn_Bus : Inport
  Bus Selector : BusSelector  OutputSignals=mach_nd
  CCDAYOD_M : Lookup_n-D  NumberOfTableDimensions=1  BreakpointsForDimension1=admireDB.aerodata_asym_ext.CCDAYOD.breakpoints.M  BreakpointsForDimension3=[5, 7]  Table=admireDB.aerodata_asym_ext.CCDAYOD.newTable  ExtrapMethod=Clip  InternalRulePriority=Speed  RndMeth=Simplest  InputSameDT=on
  Constant : Constant
  Sum : Sum  Inputs=-+|
  eoeff : Outport
  eieff : Outport  Port=2
  wires:
  Sum/1 -> eieff/1
  CCDAYOD_M/1 -> eoeff/1, Sum/1
  Constant/1 -> Sum/2
  Bus Selector/1 -> CCDAYOD_M/1  "<mach_nd>"
  AeroIn_Bus/1 -> Bus Selector/1

== system aerotest/NormalForceCoefficient/MachRegion1/Cnalfa ==
  in_bus : Inport
  Bus Selector : BusSelector  OutputSignals=AeroIn_Bus.angleOfAttack_deg,AeroIn_Bus.mach_nd,AeroIn_Bus.qacorr
  CNDEAL_DE_ALFA : Lookup_n-D  BreakpointsForDimension1=admireDB.aerodata_sym.CNDEAL.breakpoints.ALFA  BreakpointsForDimension2=admireDB.aerodata_sym.CNDEAL.breakpoints.DE  BreakpointsForDimension3=[5, 7]  Table=admireDB.aerodata_sym.CNDEAL.newTable  ExtrapMethod=Clip  InternalRulePriority=Speed  RndMeth=Simplest  InputSameDT=on
      settings: InputPortMap=u0,u1
  CNEA_QA_M : Lookup_n-D  BreakpointsForDimension1=admireDB.aerodata_sym.CNEA.breakpoints.M  BreakpointsForDimension2=admireDB.aerodata_sym.CNEA.breakpoints.QA  BreakpointsForDimension3=[5, 7]  Table=admireDB.aerodata_sym.CNEA.newTable  ExtrapMethod=Clip  InternalRulePriority=Speed  RndMeth=Simplest  InputSameDT=on
      settings: InputPortMap=u0,u1
  Constant : Constant  Value=0
  Product : Product
  Cnalfa : Outport
  wires:
  Product/1 -> Cnalfa/1
  CNDEAL_DE_ALFA/1 -> Product/1
  CNEA_QA_M/1 -> Product/2
  Bus Selector/2 -> CNEA_QA_M/1  "<mach_nd>"
  Bus Selector/3 -> CNEA_QA_M/2  "<qacorr>"
  Constant/1 -> CNDEAL_DE_ALFA/2
  Bus Selector/1 -> CNDEAL_DE_ALFA/1  "<angleOfAttack_deg>"
  in_bus/1 -> Bus Selector/1  "in_bus"

== system aerotest/NormalForceCoefficient/MachRegion1/Cnalfad ==
  in_bus : Inport
  Abs : Abs
  Bus Selector : BusSelector  OutputSignals=AeroIn_Bus.mach_nd,AeroIn_Bus.angleOfAttack_deg,AeroIn_Bus.alfad
  CNADAM_ALFA_M : Lookup_n-D  BreakpointsForDimension1=admireDB.aerodata_sym.CNADAM.breakpoints.M  BreakpointsForDimension2=admireDB.aerodata_sym.CNADAM.breakpoints.ALFA  BreakpointsForDimension3=[5, 7]  Table=admireDB.aerodata_sym.CNADAM.newTable  ExtrapMethod=Clip  InternalRulePriority=Speed  RndMeth=Simplest  InputSameDT=on
      settings: InputPortMap=u0,u1
  Product : Product
  Cnalfad : Outport
  wires:
  Abs/1 -> CNADAM_ALFA_M/2
  Bus Selector/1 -> CNADAM_ALFA_M/1  "<mach_nd>"
  Product/1 -> Cnalfad/1
  in_bus/1 -> Bus Selector/1  "in_bus"
  Bus Selector/2 -> Abs/1  "<angleOfAttack_deg>"
  CNADAM_ALFA_M/1 -> Product/1
  Bus Selector/3 -> Product/2  "<alfad>"

== system aerotest/NormalForceCoefficient/MachRegion1/Cnbasic ==
  in_bus : Inport
  Bus Selector : BusSelector  OutputSignals=AeroIn_Bus.mach_nd,AeroIn_Bus.qacorr
  CNEZERO_QA_M : Lookup_n-D  BreakpointsForDimension1=admireDB.aerodata_sym.CNEZERO.breakpoints.M  BreakpointsForDimension2=admireDB.aerodata_sym.CNEZERO.breakpoints.QA  BreakpointsForDimension3=[5, 7]  Table=admireDB.aerodata_sym.CNEZERO.newTable  ExtrapMethod=Clip  InternalRulePriority=Speed  RndMeth=Simplest  InputSameDT=on
      settings: InputPortMap=u0,u1
  CNZERO_M : Lookup_n-D  NumberOfTableDimensions=1  BreakpointsForDimension1=admireDB.aerodata_sym.CNZERO.breakpoints.M  BreakpointsForDimension3=[5, 7]  Table=admireDB.aerodata_sym.CNZERO.newTable  ExtrapMethod=Clip  InternalRulePriority=Speed  RndMeth=Simplest  InputSameDT=on
  Sum1 : Sum  Inputs=|++
  Cnbasic : Outport
  wires:
  CNEZERO_QA_M/1 -> Sum1/2
  CNZERO_M/1 -> Sum1/1
  Bus Selector/2 -> CNEZERO_QA_M/2  "<qacorr>"
  Bus Selector/1 -> CNZERO_M/1, CNEZERO_QA_M/1  "<mach_nd>"
  Sum1/1 -> Cnbasic/1
  in_bus/1 -> Bus Selector/1  "in_bus"

== system aerotest/NormalForceCoefficient/MachRegion1/Cnbeta ==
  in_bus : Inport
  Abs : Abs
  Bus Selector : BusSelector  OutputSignals=AeroIn_Bus.angleOfAttack_deg,AeroIn_Bus.dN,AeroIn_Bus.angleOfSideslip_deg
  CNBETA_DN_ALFA : Lookup_n-D  BreakpointsForDimension1=admireDB.aerodata_sym.CNBETA.breakpoints.ALFA  BreakpointsForDimension2=admireDB.aerodata_sym.CNBETA.breakpoints.DN  BreakpointsForDimension3=[5, 7]  Table=admireDB.aerodata_sym.CNBETA.newTable  ExtrapMethod=Clip  InternalRulePriority=Speed  RndMeth=Simplest  InputSameDT=on
      settings: InputPortMap=u0,u1
  CNKB_BETA : Lookup_n-D  NumberOfTableDimensions=1  BreakpointsForDimension1=admireDB.aerodata_sym.CNKB.breakpoints.BETA  BreakpointsForDimension3=[5, 7]  Table=admireDB.aerodata_sym.CNKB.newTable  ExtrapMethod=Clip  InternalRulePriority=Speed  RndMeth=Simplest  InputSameDT=on
  Product : Product
  Cnbeta : Outport
  wires:
  Product/1 -> Cnbeta/1
  CNBETA_DN_ALFA/1 -> Product/1
  CNKB_BETA/1 -> Product/2
  Abs/1 -> CNKB_BETA/1
  Bus Selector/3 -> Abs/1  "<angleOfSideslip_deg>"
  in_bus/1 -> Bus Selector/1  "in_bus"
  Bus Selector/2 -> CNBETA_DN_ALFA/2  "<dN>"
  Bus Selector/1 -> CNBETA_DN_ALFA/1  "<angleOfAttack_deg>"

== system aerotest/NormalForceCoefficient/MachRegion1/Cncai ==
  in_bus : Inport
  Bus Selector : BusSelector  OutputSignals=AeroIn_Bus.angleOfAttack_deg,AeroIn_Bus.cai
  CNCAI_CAI_ALFA : Lookup_n-D  BreakpointsForDimension1=admireDB.aerodata_sym.CNCAI.breakpoints.ALFA  BreakpointsForDimension2=admireDB.aerodata_sym.CNCAI.breakpoints.CAI  BreakpointsForDimension3=[5, 7]  Table=admireDB.aerodata_sym.CNCAI.newTable  ExtrapMethod=Clip  InternalRulePriority=Speed  RndMeth=Simplest  InputSameDT=on
      settings: InputPortMap=u0,u1
  Cncai : Outport
  wires:
  Bus Selector/1 -> CNCAI_CAI_ALFA/1  "<angleOfAttack_deg>"
  Bus Selector/2 -> CNCAI_CAI_ALFA/2  "<cai>"
  in_bus/1 -> Bus Selector/1  "in_bus"
  CNCAI_CAI_ALFA/1 -> Cncai/1

== system aerotest/NormalForceCoefficient/MachRegion1/Cndedn ==
  in_bus : Inport
  Bus Selector : BusSelector  OutputSignals=AeroIn_Bus.angleOfAttack_deg,AeroIn_Bus.dE,AeroIn_Bus.dN
  CNDNDE_ALFA_DE_DN : Lookup_n-D  NumberOfTableDimensions=3  BreakpointsForDimension1=admireDB.aerodata_sym.CNDNDE.breakpoints.ALFA  BreakpointsForDimension2=admireDB.aerodata_sym.CNDNDE.breakpoints.DE  BreakpointsForDimension3=admireDB.aerodata_sym.CNDNDE.breakpoints.DN  Table=admireDB.aerodata_sym.CNDNDE.newTable  ExtrapMethod=Clip  InternalRulePriority=Speed  RndMeth=Simplest  InputSameDT=on
      settings: InputPortMap=u0,u1,u2
  Cndedn : Outport
  wires:
  CNDNDE_ALFA_DE_DN/1 -> Cndedn/1
  Bus Selector/3 -> CNDNDE_ALFA_DE_DN/3  "<dN>"
  Bus Selector/2 -> CNDNDE_ALFA_DE_DN/2  "<dE>"
  Bus Selector/1 -> CNDNDE_ALFA_DE_DN/1  "<angleOfAttack_deg>"
  in_bus/1 -> Bus Selector/1  "in_bus"

== system aerotest/NormalForceCoefficient/MachRegion1/Cndei ==
  in_bus : Inport
  Bus Selector : BusSelector  OutputSignals=eieff,AeroIn_Bus.angleOfAttack_deg,AeroIn_Bus.dEI,AeroIn_Bus.mach_nd,AeroIn_Bus.qacorr
  CNDEAL_DE_ALFA : Lookup_n-D  BreakpointsForDimension1=admireDB.aerodata_sym.CNDEAL.breakpoints.ALFA  BreakpointsForDimension2=admireDB.aerodata_sym.CNDEAL.breakpoints.DE  BreakpointsForDimension3=[5, 7]  Table=admireDB.aerodata_sym.CNDEAL.newTable  ExtrapMethod=Clip  InternalRulePriority=Speed  RndMeth=Simplest  InputSameDT=on
      settings: InputPortMap=u0,u1
  CNDEAL_DE_ALFA1 : Lookup_n-D  BreakpointsForDimension1=admireDB.aerodata_sym.CNDEAL.breakpoints.ALFA  BreakpointsForDimension2=admireDB.aerodata_sym.CNDEAL.breakpoints.DE  BreakpointsForDimension3=[5, 7]  Table=admireDB.aerodata_sym.CNDEAL.newTable  ExtrapMethod=Clip  InternalRulePriority=Speed  RndMeth=Simplest  InputSameDT=on
      settings: InputPortMap=u0,u1
  CNEDEI_QA_M : Lookup_n-D  BreakpointsForDimension1=admireDB.aerodata_sym.CNEDEI.breakpoints.M  BreakpointsForDimension2=admireDB.aerodata_sym.CNEDEI.breakpoints.QA  BreakpointsForDimension3=[5, 7]  Table=admireDB.aerodata_sym.CNEDEI.newTable  ExtrapMethod=Clip  InternalRulePriority=Speed  RndMeth=Simplest  InputSameDT=on
      settings: InputPortMap=u0,u1
  Constant : Constant  Value=0
  Product : Product  Inputs=3
  Sum : Sum  Inputs=|+-
  Cndei : Outport
  wires:
  CNEDEI_QA_M/1 -> Product/3
  Sum/1 -> Product/2
  Bus Selector/1 -> Product/1  "<eieff>"
  Bus Selector/4 -> CNEDEI_QA_M/1  "<mach_nd>"
  Bus Selector/5 -> CNEDEI_QA_M/2  "<qacorr>"
  CNDEAL_DE_ALFA1/1 -> Sum/2
  Constant/1 -> CNDEAL_DE_ALFA1/2
  CNDEAL_DE_ALFA/1 -> Sum/1
  Bus Selector/2 -> CNDEAL_DE_ALFA/1, CNDEAL_DE_ALFA1/1  "<angleOfAttack_deg>"
  Bus Selector/3 -> CNDEAL_DE_ALFA/2  "<dEI>"
  in_bus/1 -> Bus Selector/1  "in_bus"
  Product/1 -> Cndei/1
